simulink model "robustControl"  (R2023b)
settings: Solver=VariableStepAuto  StartTime=0.0  StopTime=time(end)  RelTol=1e-3
undefined symbols (not defined in the file): DiscIntNeverNeededParam
libraries: simulink x1
settings Model: Creator=v4pal  LastModifiedBy=v4pal

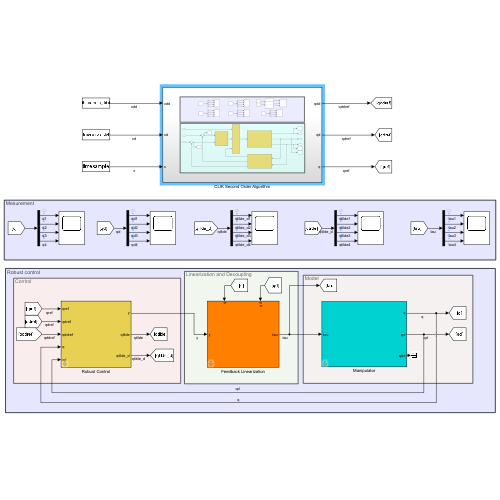
[thumbnail: Simulink's stored preview of the top-level diagram]
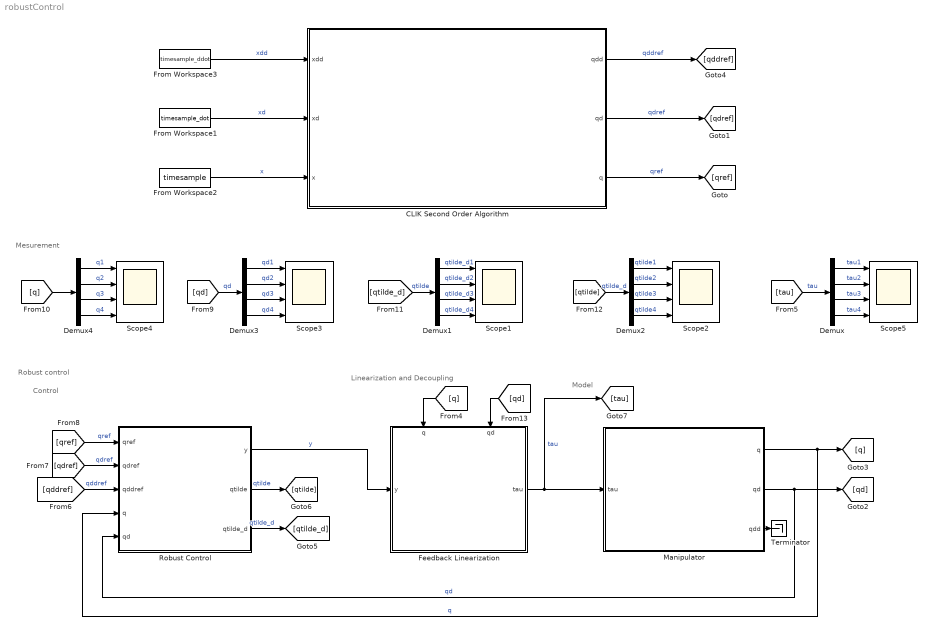
== system robustControl ==
  note: Model
  note: Linearization and Decoupling
  note: Control
  note: Robust control
  note: Mesurement
  CLIK Second Order Algorithm : Subsystem
  Demux{,1..4} (5 alike) : Demux
  Feedback Linearization : Subsystem  mask{m_load=4}
      mask prompts: m_load "Load Mass [kg]"
      settings: PortSchema="{\"entries\":[{\"content\":{\"sides\":[{\"content\":{\"connectorIds\":[\"In1\"]},\"type\":\"ConnectorPlacement.EquallySpacedRectSide\",\"uuid\":\"271cc0a6-b732-4626-ad15-944ba501bea2\"},{\"content\":{\"connectorIds\":[\"Out1\"],\"side\":\"RIGHT\"},\"type\":\"ConnectorPlacement.EquallySpacedRectSide\",\"uuid\":\"860ec51b-c9e7-4b7b-ae65-2fc3300d48f6\"},{\"content\":{\"connectorIds\":[\"In2\",\"In3\"],\"side\":\"TOP\"},\"type\":\"ConnectorPlacement.EquallySpacedRectSide\",\"uuid\":\"a378ade9-13de-47ec-a220-3e435cc4dc56\"},{\"content\":{\"side\":\"BOTTOM\"},\"type\":\"ConnectorPlacement.EquallySpacedRectSide\",\"uuid\":\"8c63b252-3c1f-48d2-9139-67a3c74d1549\"}]},\"type\":\"ConnectorPlacement.EquallySpacedConnector\",\"uuid\":\"fa57dee9-db69-4719-bb64-b991f88f74fb\"}],\"packageUris\":[\"http://schema.mathworks.com/mf0/Connector/R2020b\"],\"version\":\"1.0\"}"
      mask DialogControl DescGroupVar Prompt: Nonlinear Compensation
      mask DialogControl DescTextVar Prompt: Nonlinear compensation and decoupling block
  From Workspace1 : FromWorkspace  VariableName=timesample_dot
  From Workspace2 : FromWorkspace  VariableName=timesample
  From Workspace3 : FromWorkspace  VariableName=timesample_ddot
  Manipulator : Subsystem  mask{m_load=4, delta=10}
      mask prompts: m_load "Load Mass [kg]"; delta "Uncertainty [%]"
      mask DialogControl DescGroupVar Prompt: SCARA Dynamic Model
      mask DialogControl DescTextVar Prompt: Scara Dynamic Model with uncertainty and load mass as input.
  Robust Control : Subsystem  mask{Kd=20, Kp=200, rho=100, epsilon=0.05}
      mask prompts: Kd "Derivative Gain Kd"; Kp "Proportional Gain"
      mask DialogControl DescGroupVar Prompt: Robust Control
      mask DialogControl DescTextVar Prompt: PD controller with vers robust law
  Scope{1..5} (5 alike) : Scope  NumInputPorts=4
  Terminator : Terminator
  wires:
  [qd] -> Demux3/1  "qd"
  [qtilde_d] -> Demux1/1  "qtilde"
  [qtilde] -> Demux2/1  "qtilde_d"
  Manipulator/1(q) -> Robust Control/4(q), [q]  "q"
  Manipulator/2(qd) -> Robust Control/5(qd), [qd]  "qd"
  Manipulator/3(qdd) -> Terminator/1
  [q] -> Feedback Linearization/2(q)
  [qd] -> Feedback Linearization/3(qd)
  Feedback Linearization/1(tau) -> [tau], Manipulator/1(tau)  "tau"
  [qddref] -> Robust Control/3(qddref)  "qddref"
  [qdref] -> Robust Control/2(qdref)  "qdref"
  [qref] -> Robust Control/1(qref)  "qref"
  Robust Control/1(y) -> Feedback Linearization/1(y)  "y"
  Robust Control/3(qtilde_d) -> [qtilde_d]  "qtilde_d"
  Robust Control/2(qtilde) -> [qtilde]  "qtilde"
  [tau] -> Demux/1  "tau"
  Demux/1 -> Scope5/1  "tau1"
  Demux/2 -> Scope5/2  "tau2"
  Demux/3 -> Scope5/3  "tau3"
  Demux/4 -> Scope5/4  "tau4"
  From Workspace3/1 -> CLIK Second Order Algorithm/1(xdd)  "xdd"
  From Workspace1/1 -> CLIK Second Order Algorithm/2(xd)  "xd"
  From Workspace2/1 -> CLIK Second Order Algorithm/3(x)  "x"
  CLIK Second Order Algorithm/1(qdd) -> [qddref]  "qddref"
  CLIK Second Order Algorithm/2(qd) -> [qdref]  "qdref"
  CLIK Second Order Algorithm/3(q) -> [qref]  "qref"
  Demux1/1 -> Scope1/1  "qtilde_d1"
  Demux1/2 -> Scope1/2  "qtilde_d2"
  Demux1/3 -> Scope1/3  "qtilde_d3"
  Demux1/4 -> Scope1/4  "qtilde_d4"
  Demux2/4 -> Scope2/4  "qtilde4"
  Demux2/3 -> Scope2/3  "qtilde3"
  Demux2/2 -> Scope2/2  "qtilde2"
  Demux2/1 -> Scope2/1  "qtilde1"
  [q] -> Demux4/1
  Demux3/1 -> Scope3/1  "qd1"
  Demux3/2 -> Scope3/2  "qd2"
  Demux3/3 -> Scope3/3  "qd3"
  Demux3/4 -> Scope3/4  "qd4"
  Demux4/4 -> Scope4/4  "q4"
  Demux4/3 -> Scope4/3  "q3"
  Demux4/2 -> Scope4/2  "q2"
  Demux4/1 -> Scope4/1  "q1"

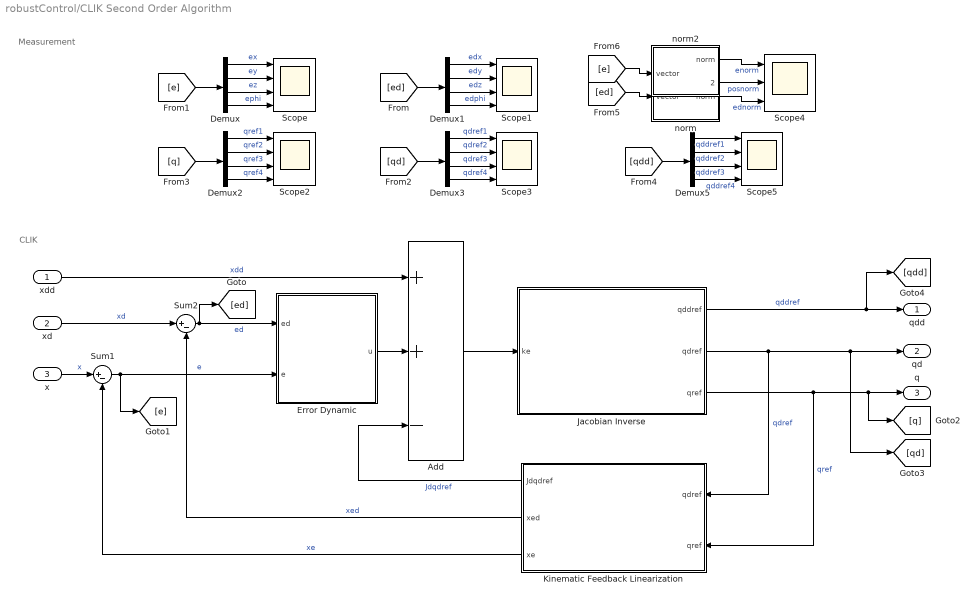
== system robustControl/CLIK Second Order Algorithm ==
  note: CLIK
  note: Measurement
  xdd : Inport
  xd : Inport  Port=2
  x : Inport  Port=3
  Add : Sum  Inputs=++-
  Demux{,1..3,5} (5 alike) : Demux
  Error Dynamic : Subsystem  mask{Kd1=50, Kd2=50, Kd3=50, Kd4=50, Kp1=500, Kp2=500, Kp3=500, Kp4=500, Ki=0}
  Jacobian Inverse : Subsystem
  Kinematic Feedback Linearization : Subsystem
  Scope{,1..3,5} (5 alike) : Scope  NumInputPorts=4
  Scope4 : Scope  NumInputPorts=3
  Sum1 : Sum  Inputs=|+-
  Sum2 : Sum  Inputs=|+-
  norm : Subsystem
  norm2 : Subsystem
  qdd : Outport
  qd : Outport  Port=2
  q : Outport  Port=3
  wires:
  Sum1/1 -> [e], Error Dynamic/2(e)  "e"
  Jacobian Inverse/2(qdref) -> [qd], qd/1, Kinematic Feedback Linearization/1(qdref)  "qdref"
  Sum2/1 -> Error Dynamic/1(ed), [ed]  "ed"
  Add/1 -> Jacobian Inverse/1(ke)
  x/1 -> Sum1/1  "x"
  Jacobian Inverse/3(qref) -> [q], q/1, Kinematic Feedback Linearization/2(qref)  "qref"
  Kinematic Feedback Linearization/1(Jdqdref) -> Add/3  "Jdqdref"
  Kinematic Feedback Linearization/3(xe) -> Sum1/2  "xe"
  Kinematic Feedback Linearization/2(xed) -> Sum2/2  "xed"
  xd/1 -> Sum2/1  "xd"
  Jacobian Inverse/1(qddref) -> [qdd], qdd/1  "qddref"
  xdd/1 -> Add/1  "xdd"
  [ed] -> Demux1/1
  [e] -> Demux/1
  Demux/1 -> Scope/1  "ex"
  Demux/2 -> Scope/2  "ey"
  Demux/3 -> Scope/3  "ez"
  Demux/4 -> Scope/4  "ephi"
  Demux1/1 -> Scope1/1  "edx"
  Demux1/2 -> Scope1/2  "edy"
  Demux1/3 -> Scope1/3  "edz"
  Demux1/4 -> Scope1/4  "edphi"
  Demux3/4 -> Scope3/4  "qdref4"
  Demux3/3 -> Scope3/3  "qdref3"
  Demux3/2 -> Scope3/2  "qdref2"
  Demux3/1 -> Scope3/1  "qdref1"
  Demux2/4 -> Scope2/4  "qref4"
  Demux2/3 -> Scope2/3  "qref3"
  Demux2/2 -> Scope2/2  "qref2"
  Demux2/1 -> Scope2/1  "qref1"
  [q] -> Demux2/1
  [qd] -> Demux3/1
  [qdd] -> Demux5/1
  Demux5/1 -> Scope5/1  "qddref1"
  Demux5/2 -> Scope5/2  "qddref2"
  Demux5/3 -> Scope5/3  "qddref3"
  Demux5/4 -> Scope5/4  "qddref4"
  [e] -> norm2/1(vector)
  norm2/1(norm) -> Scope4/1  "enorm"
  norm/1(norm) -> Scope4/3  "ednorm"
  [ed] -> norm/1(vector)
  Error Dynamic/1(u) -> Add/2
  norm2/2(posnorm) -> Scope4/2  "posnorm"

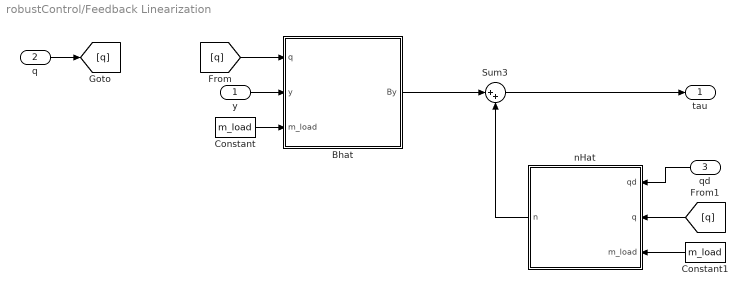
== system robustControl/Feedback Linearization ==
  y : Inport
  q : Inport  Port=2
  qd : Inport  Port=3
  Bhat : MATLAB Function  TreatAsAtomicUnit=on
  Constant : Constant  Value=m_load
  Constant1 : Constant  Value=m_load
  Sum3 : Sum  Inputs=|++
  nHat : MATLAB Function  TreatAsAtomicUnit=on
  tau : Outport
  wires:
  nHat/1(n) -> Sum3/2
  [q] -> nHat/2(q)
  qd/1 -> nHat/1(qd)
  Sum3/1 -> tau/1
  Bhat/1(By) -> Sum3/1
  y/1 -> Bhat/2(y)
  Constant/1 -> Bhat/3(m_load)
  Constant1/1 -> nHat/3(m_load)
  q/1 -> [q]
  [q] -> Bhat/1(q)

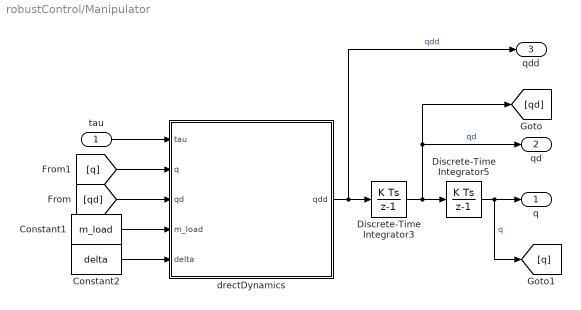
== system robustControl/Manipulator ==
  tau : Inport
  Constant1 : Constant  Value=m_load
  Constant2 : Constant  Value=delta
  Discrete-Time Integrator3 : DiscreteIntegrator  InitialCondition=[0; 0; 0; 0]  SampleTime=0.001  ICPrevOutput=DiscIntNeverNeededParam  ICPrevScaledInput=DiscIntNeverNeededParam
  Discrete-Time Integrator5 : DiscreteIntegrator  InitialCondition=[-1.5706; 0.7851; 0.5000; -0.7855]  SampleTime=0.001  ICPrevOutput=DiscIntNeverNeededParam  ICPrevScaledInput=DiscIntNeverNeededParam
  drectDynamics : MATLAB Function  TreatAsAtomicUnit=on
  q : Outport
  qd : Outport  Port=2
  qdd : Outport  Port=3
  wires:
  tau/1 -> drectDynamics/1(tau)
  Constant1/1 -> drectDynamics/4(m_load)
  drectDynamics/1(qdd) -> qdd/1, Discrete-Time Integrator3/1  "qdd"
  Discrete-Time Integrator3/1 -> [qd], qd/1, Discrete-Time Integrator5/1  "qd"
  Discrete-Time Integrator5/1 -> [q], q/1  "q"
  [qd] -> drectDynamics/3(qd)
  [q] -> drectDynamics/2(q)
  Constant2/1 -> drectDynamics/5(delta)

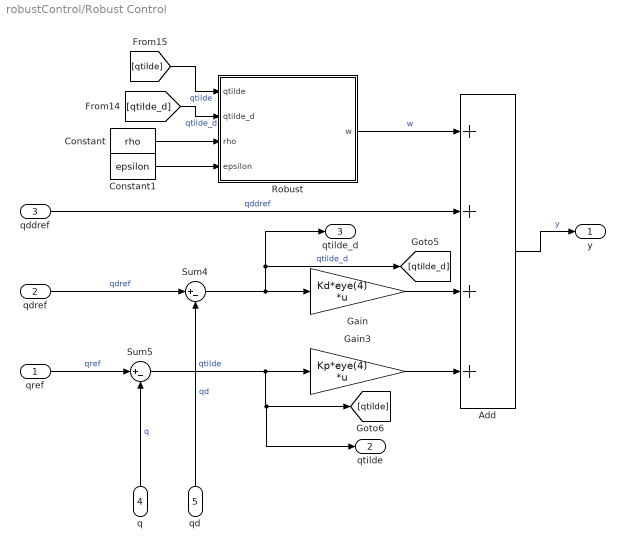
== system robustControl/Robust Control ==
  qref : Inport
  qdref : Inport  Port=2
  qddref : Inport  Port=3
  q : Inport  Port=4
  qd : Inport  Port=5
  Add : Sum  Inputs=++++
  Constant : Constant  Value=rho
  Constant1 : Constant  Value=epsilon
  Gain : Gain  Gain=Kd*eye(4)  Multiplication=Matrix(K*u)
  Gain3 : Gain  Gain=Kp*eye(4)  Multiplication=Matrix(K*u)
  Robust : MATLAB Function  TreatAsAtomicUnit=on
  Sum4 : Sum  Inputs=|+-
  Sum5 : Sum  Inputs=|+-
  y : Outport
  qtilde : Outport  Port=2
  qtilde_d : Outport  Port=3
  wires:
  Gain/1 -> Add/3
  Sum4/1 -> qtilde_d/1, [qtilde_d], Gain/1  "qtilde_d"
  Gain3/1 -> Add/4
  Sum5/1 -> Gain3/1, qtilde/1, [qtilde]  "qtilde"
  Robust/1(w) -> Add/1  "w"
  [qtilde_d] -> Robust/2(qtilde_d)  "qtilde_d"
  [qtilde] -> Robust/1(qtilde)  "qtilde"
  qdref/1 -> Sum4/1  "qdref"
  qddref/1 -> Add/2  "qddref"
  q/1 -> Sum5/2  "q"
  qref/1 -> Sum5/1  "qref"
  qd/1 -> Sum4/2  "qd"
  Add/1 -> y/1  "y"
  Constant/1 -> Robust/3(rho)
  Constant1/1 -> Robust/4(epsilon)

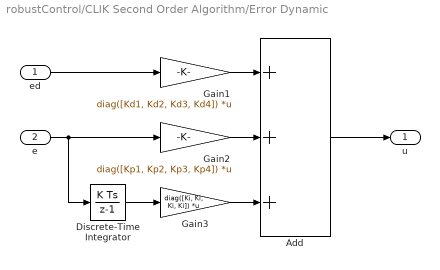
== system robustControl/CLIK Second Order Algorithm/Error Dynamic ==
  ed : Inport
  e : Inport  Port=2
  Add : Sum  Inputs=+++
  Discrete-Time Integrator : DiscreteIntegrator  SampleTime=0.001  ICPrevOutput=DiscIntNeverNeededParam  ICPrevScaledInput=DiscIntNeverNeededParam
  Gain1 : Gain  Gain=diag([Kd1, Kd2, Kd3, Kd4])  Multiplication=Matrix(K*u)
  Gain2 : Gain  Gain=diag([Kp1, Kp2, Kp3, Kp4])  Multiplication=Matrix(K*u)
  Gain3 : Gain  Gain=diag([Ki, Ki, Ki, Ki])  Multiplication=Matrix(K*u)
  u : Outport
  wires:
  Gain2/1 -> Add/2
  Gain1/1 -> Add/1
  ed/1 -> Gain1/1
  e/1 -> Discrete-Time Integrator/1, Gain2/1
  Gain3/1 -> Add/3
  Discrete-Time Integrator/1 -> Gain3/1
  Add/1 -> u/1

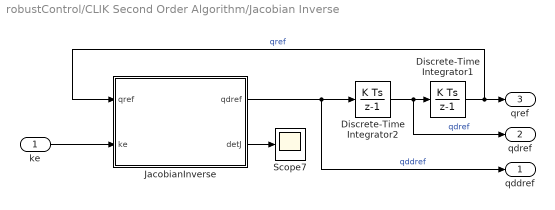
== system robustControl/CLIK Second Order Algorithm/Jacobian Inverse ==
  ke : Inport
  Discrete-Time Integrator1 : DiscreteIntegrator  InitialCondition=[-1.5706; 0.7851; 0.5000; -0.7855]  SampleTime=0.001  ICPrevOutput=DiscIntNeverNeededParam  ICPrevScaledInput=DiscIntNeverNeededParam
  Discrete-Time Integrator2 : DiscreteIntegrator  InitialCondition=[0; 0; 0; 0]  SampleTime=0.001  ICPrevOutput=DiscIntNeverNeededParam  ICPrevScaledInput=DiscIntNeverNeededParam
  JacobianInverse : MATLAB Function  TreatAsAtomicUnit=on
  Scope7 : Scope
  qddref : Outport
  qdref : Outport  Port=2
  qref : Outport  Port=3
  wires:
  JacobianInverse/2(detJ) -> Scope7/1
  Discrete-Time Integrator2/1 -> qdref/1, Discrete-Time Integrator1/1  "qdref"
  JacobianInverse/1(qdref) -> qddref/1, Discrete-Time Integrator2/1  "qddref"
  Discrete-Time Integrator1/1 -> JacobianInverse/1(qref), qref/1  "qref"
  ke/1 -> JacobianInverse/2(ke)

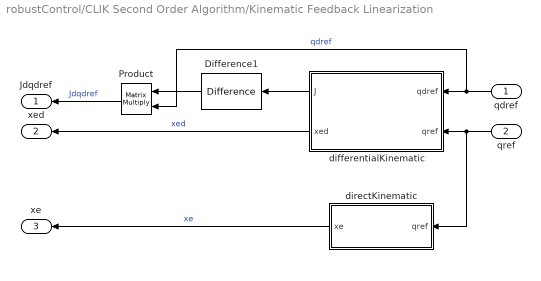
== system robustControl/CLIK Second Order Algorithm/Kinematic Feedback Linearization ==
  qdref : Inport
  qref : Inport  Port=2
  Difference1 : simulink/Discrete/Difference  ICPrevInput=0.0  OutMin=[]  OutMax=[]  OutDataType=fixdt(1, 16)  OutScaling=2^-10  DoSatur=off
  Product : Product  Multiplication=Matrix(*)
  differentialKinematic : MATLAB Function  TreatAsAtomicUnit=on
  directKinematic : MATLAB Function  TreatAsAtomicUnit=on
  Jdqdref : Outport
  xed : Outport  Port=2
  xe : Outport  Port=3
  wires:
  Product/1 -> Jdqdref/1  "Jdqdref"
  Difference1/1 -> Product/1
  qref/1 -> directKinematic/1(qref), differentialKinematic/2(qref)
  differentialKinematic/2(xed) -> xed/1  "xed"
  qdref/1 -> Product/2, differentialKinematic/1(qdref)  "qdref"
  differentialKinematic/1(J) -> Difference1/1
  directKinematic/1(xe) -> xe/1  "xe"

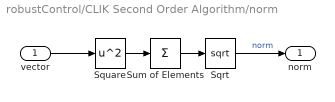
== system robustControl/CLIK Second Order Algorithm/norm ==
  vector : Inport
  Sqrt : Sqrt
  Square : Math  Operator=square
  Sum of Elements : Sum  Inputs=+
  norm : Outport
  wires:
  Sqrt/1 -> norm/1  "norm"
  vector/1 -> Square/1
  Sum of Elements/1 -> Sqrt/1
  Square/1 -> Sum of Elements/1

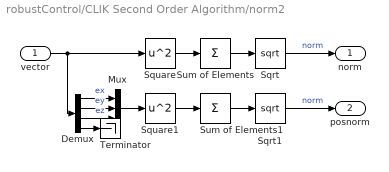
== system robustControl/CLIK Second Order Algorithm/norm2 ==
  vector : Inport
  Demux : Demux
  Mux : Mux  Inputs=3
  Sqrt : Sqrt
  Sqrt1 : Sqrt
  Square : Math  Operator=square
  Square1 : Math  Operator=square
  Sum of Elements : Sum  Inputs=+
  Sum of Elements1 : Sum  Inputs=+
  Terminator : Terminator
  norm : Outport
  posnorm : Outport  Port=2
  wires:
  Square/1 -> Sum of Elements/1
  Sum of Elements/1 -> Sqrt/1
  vector/1 -> Demux/1, Square/1
  Sqrt/1 -> norm/1  "norm"
  Sqrt1/1 -> posnorm/1  "norm"
  Sum of Elements1/1 -> Sqrt1/1
  Square1/1 -> Sum of Elements1/1
  Mux/1 -> Square1/1
  Demux/1 -> Mux/1  "ex"
  Demux/2 -> Mux/2  "ey"
  Demux/3 -> Mux/3  "ez"
  Demux/4 -> Terminator/1

== matlab function robustControl/CLIK Second Order Algorithm/Kinematic Feedback Linearization/differentialKinematic ==
  data: qdref input; J output; qref input; xed output
function [J, xed] = Jacobian(qdref, qref)

    % Init the SCARA manipulator parameters
    a1 = .5; a2 = .5;
    theta1 = qref(1,:); theta2 = qref(2,:);
    
    %% Geometric Jacobian Matrix
    Ja = [-a1*sin(theta1) - a2*sin(theta1 + theta2), - a2*sin(theta1 + theta2), 0, 0;
        a1*cos(theta1) + a2*cos(theta1 + theta2), a2*cos(theta1 + theta2), 0, 0;
        0, 0, -1, 0;
        1, 1, 0, -1;];

    % Vx = Jx1 * qd1 + Jx2 * qd2 +Jx3 * qd3;
    % Vy = Jy1 * qd1 + Jy2 * qd2 +Jy3 * qd3;
    % Vz = Jz1 * qd1 + Jz2 * qd2 +Jz3 * qd3;
    
    %J = Ja(1:3,1:3);
    J = Ja;

    %% Calculation of xe_dot
    xed = J * qdref;

end

== matlab function robustControl/CLIK Second Order Algorithm/Kinematic Feedback Linearization/directKinematic ==
  data: qref input; xe output
function xe = directKinematic(qref)
    
    %% Init the SCARA manipulator parameters and Joint variables
    a1 = .5; a2 = .5; d0 = 1;
    theta1 = qref(1,:); theta2 = qref(2,:); d3 = qref(3,:); theta4 = qref(4,:);

    %% Forward Kinematics link for the SCARA
    k = [a1*cos(theta1) + a2*cos(theta1 + theta2);
        a1*sin(theta1) + a2*sin(theta1 + theta2);
        d0 - d3;
        theta1 + theta2 - theta4;];

    xe = k;

end

== matlab function robustControl/Feedback Linearization/nHat ==
  data: qd input; q input; n output; m_load input
function n = nHat(qd,q,m_load)
    
    q1 = q(1,:);
    q2 = q(2,:);
    q3 = q(3,:);
    qd1 = qd(1,:);
    qd2 = qd(2,:);
    
    %% parametri
    a1 = 0.5;
    a2 = 0.5;
    d0 = 1;
    
    ml1 = 20;
    ml2 = 20;
    ml3 = 10;
    l1 = 0.25;
    l2 = 0.25;
    kr1 = 1;
    kr2 = 1;
    kr3 = 50;
    kr4 = 20;
    Fm1 =  0.00005;
    Fm2 =  0.00005;
    Fm3 = 0.01;
    Fm4 = 0.005;
    
    %% calcolo p pl z
    p0 = [0 ; 0 ; d0];
    p1 = [a1*cos(q1) ; a1*sin(q1) ; d0];
    p2 = [a1*cos(q1) + a2*cos(q1+q2) ; a1*sin(q1) + a2*sin(q1+q2) ; d0];
    p3 = p2 - [0 ; 0 ; q3];
    p4 = p3;
    pl1 = [l1*cos(q1) ; l1*sin(q1) ; d0];
    pl2 = [a1*cos(q1) + l2*cos(q1+q2) ; a1*sin(q1) + l2*sin(q1+q2) ; d0];
    pl3 = p3; % ????
    pl4 = p4; % 
    z0 = [0 0 1]';
    z1 = [0 0 1]';
    z2 = [0 0 -1]';
    z3 = [0 0 -1]';
    
    %% calcolo JPl JOl JOm
    JP_l1 = [cross(z0,pl1-p0) zeros(3,3)];
    JP_l2 = [cross(z0,pl2-p0) cross(z1,pl2-p1) zeros(3,2)];
    JP_l3 = [cross(z0,pl3-p0) cross(z1,pl3-p1) z2 zeros(3,1)]; 
    JP_l4 = [cross(z0,pl4-p0) cross(z1,pl4-p1) z2 cross(z3,pl4-p3)]; %m4=mload

    %% Contributo di gravità sull'iesimo link.(Formula 7.39)
    g0 = [0 0 -9.81]';
    g1 = - (ml1*g0'*JP_l1(:,1) + ml2*g0'*JP_l2(:,1) + ml3*g0'*JP_l3(:,1) + m_load*g0'*JP_l4(:,1));
    g2 = - (ml1*g0'*JP_l1(:,2) + ml2*g0'*JP_l2(:,2) + ml3*g0'*JP_l3(:,2) + m_load*g0'*JP_l4(:,2));
    g3 = - (ml1*g0'*JP_l1(:,3) + ml2*g0'*JP_l2(:,3) + ml3*g0'*JP_l3(:,3) + m_load*g0'*JP_l4(:,3));
    g4 = - (ml1*g0'*JP_l1(:,4) + ml2*g0'*JP_l2(:,4) + ml3*g0'*JP_l3(:,4) + m_load*g0'*JP_l4(:,4));
    g = [g1 g2 g3 g4]';
    
    %% Contributo di accelerazione C
    C = [-a1*qd2*sin(q2)*(a2*m_load + a2*ml3 + l2*ml2), -a1*sin(q2)*(qd1 + qd2)*(a2*m_load + a2*ml3 + l2*ml2), 0, 0;
          a1*qd1*sin(q2)*(a2*m_load + a2*ml3 + l2*ml2),  0, 0, 0;
          0, 0, 0, 0;
          0, 0, 0, 0]; 
    
    %% Attrito viscoso al manipolatore
    Fv = diag([kr1^2*Fm1 kr2^2*Fm2 kr3^2*Fm3 kr4^2*Fm4]);

    n = C*qd + Fv*qd + g;

end

== matlab function robustControl/Feedback Linearization/Bhat ==
  data: q input; By output; y input; m_load input
function By = Bhat(q,y,m_load)
    
    q1 = q(1,:);
    q2 = q(2,:);
    q3 = q(3,:);
    q4 = q(4,:);
    
    %% parametri
    a1 = 0.5;
    a2 = 0.5;
    d0 = 1;
    
    ml1 = 20;
    ml2 = 20;
    ml3 = 10;
    Il1 = 4;
    Il2 = 4;
    Il4 = 1;
    Im1 = 0.01;
    Im2 = 0.01;
    Im3 = 0.005;
    Im4 = 0.001;
    l1 = 0.25;
    l2 = 0.25;
    kr1 = 1;
    kr2 = 1;
    kr3 = 50;
    kr4 = 20;
    Fm1 =  0.00005;
    Fm2 =  0.00005;
    Fm3 = 0.01;
    Fm4 = 0.005;
    
    %% calcolo p pl z
    p0 = [0 ; 0 ; d0];
    p1 = [a1*cos(q1) ; a1*sin(q1) ; d0];
    p2 = [a1*cos(q1) + a2*cos(q1+q2) ; a1*sin(q1) + a2*sin(q1+q2) ; d0];
    p3 = p2 - [0 ; 0 ; q3];
    p4 = p3;
    pl1 = [l1*cos(q1) ; l1*sin(q1) ; d0];
    pl2 = [a1*cos(q1) + l2*cos(q1+q2) ; a1*sin(q1) + l2*sin(q1+q2) ; d0];
    pl3 = p3; % ????
    pl4 = p4; % 
    z0 = [0 0 1]';
    z1 = [0 0 1]';
    z2 = [0 0 -1]';
    z3 = [0 0 -1]';
    
    %% calcolo JPl JOl JOm
    JP_l1 = [cross(z0,pl1-p0) zeros(3,3)];
    JP_l2 = [cross(z0,pl2-p0) cross(z1,pl2-p1) zeros(3,2)];
    JP_l3 = [cross(z0,pl3-p0) cross(z1,pl3-p1) z2 zeros(3,1)]; 
    JP_l4 = [cross(z0,pl4-p0) cross(z1,pl4-p1) z2 cross(z3,pl4-p3)]; %m4=mload
    
    JO_l1 = [z0 zeros(3,3)];
    JO_l2 = [z0 z1 zeros(3,2)];
    %JO_l3 = [z0 z1 zeros(3,2)]; Il3=0
    JO_l4 = [z0 z1 zeros(3,1) z3];
    
    %assumo che zm1=z0, zm2=z1, zm3=-z2, zm4=z3-->si trova sul giunto
    JO_m1 = JO_l1;
    JO_m1(:,1) = kr1*z0;
    JO_m2 = JO_l2;  
    JO_m2(:,2) = kr2*z1;
    JO_m3 = [z0 z1 zeros(3,2)]; 
    JO_m3(:,3) = kr3*z2;
    JO_m4 = JO_l4;
    JO_m4(:,4) = kr4*z3;
    
    %% Matrice d'Inerzia B (eq 7.32)
    B1 = ml1*(JP_l1'*JP_l1) + Il1*(JO_l1'*JO_l1) + Im1*(JO_m1'*JO_m1) ; 
    B2 = ml2*(JP_l2'*JP_l2) + Il2*(JO_l2'*JO_l2) + Im2*(JO_m2'*JO_m2) ; 
    B3 = ml3*(JP_l3'*JP_l3) + 0 + Im3*(JO_m3'*JO_m3) ; %Il3=0
    B4 = m_load*(JP_l4'*JP_l4) + Il4*(JO_l4'*JO_l4) + Im4*(JO_m4'*JO_m4) ; 
    B = B1 + B2 + B3 + B4;
    
    By = B * y;

end

== matlab function robustControl/CLIK Second Order Algorithm/Jacobian Inverse/JacobianInverse ==
  data: qref input; ke input; qdref output; detJ output
function [qdref, detJ] = inverseJacobian(qref, ke) % q = [theta1; theta2]

    % Init the SCARA manipulator parameters
    a1 = .5; a2 = .5;

    theta1 = qref(1,:); theta2 = qref(2,:);
    %% Geometric Jacobian Matrix
    J = [-a1*sin(theta1) - a2*sin(theta1 + theta2), - a2*sin(theta1 + theta2), 0, 0;
        a1*cos(theta1) + a2*cos(theta1 + theta2), a2*cos(theta1 + theta2), 0, 0;
        0, 0, -1, 0;
        1, 1, 0, -1;];

    % Vx = Jx1 * qd1 + Jx2 * qd2 +Jx3 * qd3;
    % Vy = Jy1 * qd1 + Jy2 * qd2 +Jy3 * qd3;
    % Vz = Jz1 * qd1 + Jz2 * qd2 +Jz3 * qd3;
    
    %J = J(1:3,1:3);
    
    detJ = det(J);
    % Calculate the inverse of the Jacobian matrix
    J_inv = inv(J);

    % Calculate joint velocities
    qdref = J_inv * ke;

end

== matlab function robustControl/Manipulator/drectDynamics ==
  data: tau input; q input; qdd output; qd input; m_load input; delta input
function qdd = directDynamics(tau,q,qd,m_load,delta)

%% Needed joint position and velocity
q1 = q(1,:);
q2 = q(2,:);
q3 = q(3,:);
qd1 = qd(1,:);
qd2 = qd(2,:);

%% Dynamic Parameters
a1 = 0.5; a2 = 0.5; d0 = 1;
ml1 = 20; ml2 = 20; ml3 = 10;
Il1 = 4; Il2 = 4; Il4 = 1;
Im1 = 0.01; Im2 = 0.01; Im3 = 0.005; Im4 = 0.001;
l1 = 0.25; l2 = 0.25;
kr1 = 1; kr2 = 1; kr3 = 50; kr4 = 20;
Fm1 =  0.00005; Fm2 =  0.00005; Fm3 = 0.01; Fm4 = 0.005;

%% Adding Uncertainty
delta = delta/100; % converting from percentage 
ml1 = ml1 + delta*ml1; ml2 = ml2 + delta*ml2; ml3 = ml3 + delta*ml3;
Il1 = Il1 + delta*Il1; Il2 = Il2 + delta*Il2; Il4 = Il4 + delta*Il4;
l1 = l1 + delta*l1; l2 = l2 + delta*l2;
Fm1 = Fm1 + delta*Fm1;


%% Position vector and z unit vector 
p0 = [0 ; 0 ; d0];
p1 = [a1*cos(q1) ; a1*sin(q1) ; d0];
p2 = [a1*cos(q1) + a2*cos(q1+q2) ; a1*sin(q1) + a2*sin(q1+q2) ; d0];
p3 = p2 - [0 ; 0 ; q3];
p4 = p3;
pl1 = [l1*cos(q1) ; l1*sin(q1) ; d0];
pl2 = [a1*cos(q1) + l2*cos(q1+q2) ; a1*sin(q1) + l2*sin(q1+q2) ; d0];
pl3 = p3; % ????
pl4 = p4; % 
z0 = [0 0 1]';
z1 = [0 0 1]';
z2 = [0 0 -1]';
z3 = [0 0 -1]';

%% Positional and orientation jacobian of links (JPl JOl JOm)
JP_l1 = [cross(z0,pl1-p0) zeros(3,3)];
JP_l2 = [cross(z0,pl2-p0) cross(z1,pl2-p1) zeros(3,2)];
JP_l3 = [cross(z0,pl3-p0) cross(z1,pl3-p1) z2 zeros(3,1)]; 
JP_l4 = [cross(z0,pl4-p0) cross(z1,pl4-p1) z2 cross(z3,pl4-p3)]; %m4=mload

JO_l1 = [z0 zeros(3,3)];
JO_l2 = [z0 z1 zeros(3,2)];
%JO_l3 = [z0 z1 zeros(3,2)]; Il3=0
JO_l4 = [z0 z1 zeros(3,1) z3];

%assuming zm1=z0, zm2=z1, zm3=-z2, zm4=z3-->it's on the joint
JO_m1 = JO_l1;
JO_m1(:,1) = kr1*z0;
JO_m2 = JO_l2;  
JO_m2(:,2) = kr2*z1;
JO_m3 = [z0 z1 zeros(3,2)]; 
JO_m3(:,3) = kr3*z2;
JO_m4 = JO_l4;
JO_m4(:,4) = kr4*z3;

%% Inertia matrix B (eq 7.32)
B1 = ml1*(JP_l1'*JP_l1) + Il1*(JO_l1'*JO_l1) + Im1*(JO_m1'*JO_m1) ; 
B2 = ml2*(JP_l2'*JP_l2) + Il2*(JO_l2'*JO_l2) + Im2*(JO_m2'*JO_m2) ; 
B3 = ml3*(JP_l3'*JP_l3) + 0 + Im3*(JO_m3'*JO_m3) ; %Il3=0
B4 = m_load*(JP_l4'*JP_l4) + Il4*(JO_l4'*JO_l4) + Im4*(JO_m4'*JO_m4) ; 
B = B1 + B2 + B3 + B4;

%% Gravity forces(Formula 7.39)
g0 = [0 0 -9.81]';
g1 = - (ml1*g0'*JP_l1(:,1) + ml2*g0'*JP_l2(:,1) + ml3*g0'*JP_l3(:,1) + m_load*g0'*JP_l4(:,1));
g2 = - (ml1*g0'*JP_l1(:,2) + ml2*g0'*JP_l2(:,2) + ml3*g0'*JP_l3(:,2) + m_load*g0'*JP_l4(:,2));
g3 = - (ml1*g0'*JP_l1(:,3) + ml2*g0'*JP_l2(:,3) + ml3*g0'*JP_l3(:,3) + m_load*g0'*JP_l4(:,3));
g4 = - (ml1*g0'*JP_l1(:,4) + ml2*g0'*JP_l2(:,4) + ml3*g0'*JP_l3(:,4) + m_load*g0'*JP_l4(:,4));
g = [g1 g2 g3 g4]';

%% Coriolis matrix C
C = [-a1*qd2*sin(q2)*(a2*m_load + a2*ml3 + l2*ml2), -a1*sin(q2)*(qd1 + qd2)*(a2*m_load + a2*ml3 + l2*ml2), 0, 0;
      a1*qd1*sin(q2)*(a2*m_load + a2*ml3 + l2*ml2),  0, 0, 0;
      0, 0, 0, 0;
      0, 0, 0, 0]; 

%% Friction
Fv = diag([kr1^2*Fm1 kr2^2*Fm2 kr3^2*Fm3 kr4^2*Fm4]);

%% Acceleration computation
qdd = inv(B)*(tau - C*qd -Fv*qd -g);

end

== matlab function robustControl/Robust Control/Robust ==
  data: qtilde input; qtilde_d input; w output; rho input; epsilon input
function w = vers(qtilde, qtilde_d, rho, epsilon)
    
    D = [zeros(4,4); eye(4)];
    Q = eye(8);
    xi = [qtilde; qtilde_d];

    z = D'*Q*xi;

    if norm(z) >= epsilon   
       w = rho * z / norm(z);
    else 
        w = rho * z / epsilon;
    end
    
end
